simulink library "HIL_UDP_lib"  (Simulink 8.1)
settings: Solver=ode45  StartTime=0.0  StopTime=10.0  RelTol=1e-3
undefined symbols (not defined in the file): generic_ethernet_cb
libraries: HIL_UDP_lib x9, rtlab x2, simulink x2, opal_lib x1
settings Model: Creator=ch24070  LastModifiedBy=re25624

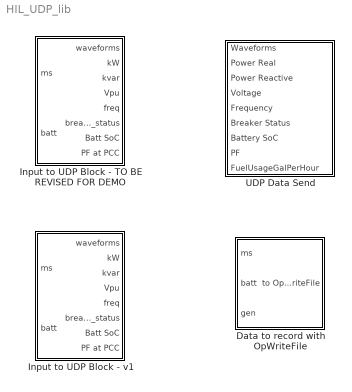
== system HIL_UDP_lib ==
  Data to record with OpWriteFile : Subsystem
  Input to UDP Block - TO BE REVISED FOR DEMO : Subsystem
  Input to UDP Block - v1 : Subsystem
  UDP Data Send : Subsystem

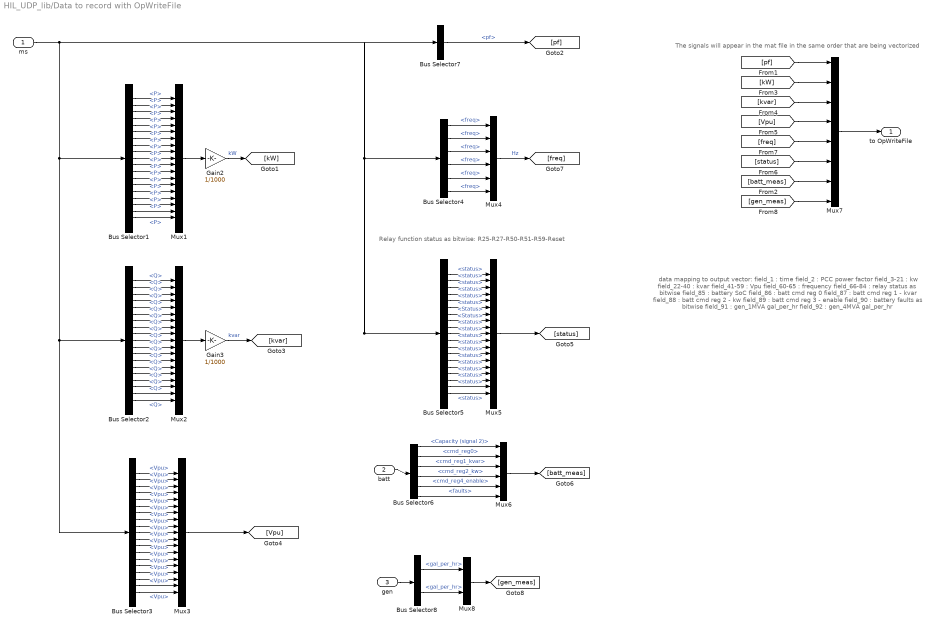
== system HIL_UDP_lib/Data to record with OpWriteFile ==
  note: The signals will appear in the mat file in the same order that are being vectorized
  note: Relay function status as bitwise:
      | R25-R27-R50-R51-R59-Reset
  note: data mapping to output vector:
      | field_1 : time
      | field_2 : PCC power factor
      | field_3-21 : kw
      | field_22-40 : kvar
      | field_41-59 : Vpu
      | field_60-65 : frequency
      | field_66-84 : relay status as bitwise
      | field_85 : battery SoC
      | field_86 : batt cmd reg 0
      | field_87 : batt cmd reg 1 - kvar
      | field_88 : batt cmd reg 2 - kw
      | field_89 : batt cmd reg 3 - enable
      | field_90 : battery faults as bitwise
      | field_91 : gen_1MVA gal_per_hr
      | field_92 : gen_4MVA gal_per_hr
  ms : Inport
  batt : Inport  Port=2
  gen : Inport  Port=3
  Bus Selector1 : BusSelector  OutputSignals=SEL_787_Relay1.m.P,SEL_787_Relay2.m.P,SEL_787_Relay3.m.P,SEL_787_Relay4.m.P,SEL_787_Relay5.m.P,SEL_787_Relay6.m.P,SEL_787_Relay7.P,SEL_787_Relay8.P,SEL_787_Relay9.m.P,SEL_787_Relay10.m.P,SEL_787_Relay11.m.P,SEL_787_Relay12.m.P,SEL_787_Relay13.m.P,SEL_787_Relay14.m.P,SEL_787_Relay15.m.P,SEL_787_Relay16.m.P,SEL_787_Relay17.m.P,SEL_787_Relay18.m.P,SEL_787_Relay19.m.P
  Bus Selector2 : BusSelector  OutputSignals=SEL_787_Relay1.m.Q,SEL_787_Relay2.m.Q,SEL_787_Relay3.m.Q,SEL_787_Relay4.m.Q,SEL_787_Relay5.m.Q,SEL_787_Relay6.m.Q,SEL_787_Relay7.Q,SEL_787_Relay8.Q,SEL_787_Relay9.m.Q,SEL_787_Relay10.m.Q,SEL_787_Relay11.m.Q,SEL_787_Relay12.m.Q,SEL_787_Relay13.m.Q,SEL_787_Relay14.m.Q,SEL_787_Relay15.m.Q,SEL_787_Relay16.m.Q,SEL_787_Relay17.m.Q,SEL_787_Relay18.m.Q,SEL_787_Relay19.m.Q
  Bus Selector3 : BusSelector  OutputSignals=SEL_787_Relay1.m.Vpu,SEL_787_Relay2.m.Vpu,SEL_787_Relay3.m.Vpu,SEL_787_Relay4.m.Vpu,SEL_787_Relay5.m.Vpu,SEL_787_Relay6.m.Vpu,SEL_787_Relay7.Vpu,SEL_787_Relay8.Vpu,SEL_787_Relay9.m.Vpu,SEL_787_Relay10.m.Vpu,SEL_787_Relay11.m.Vpu,SEL_787_Relay12.m.Vpu,SEL_787_Relay13.m.Vpu,SEL_787_Relay14.m.Vpu,SEL_787_Relay15.m.Vpu,SEL_787_Relay16.m.Vpu,SEL_787_Relay17.m.Vpu,SEL_787_Relay18.m.Vpu,SEL_787_Relay19.m.Vpu
  Bus Selector4 : BusSelector  OutputSignals=SEL_787_Relay1.m.freq,SEL_787_Relay3.m.freq,SEL_787_Relay7.freq,SEL_787_Relay8.freq,SEL_787_Relay13.m.freq,SEL_787_Relay17.m.freq
  Bus Selector5 : BusSelector  OutputSignals=SEL_787_Relay1.m.status,SEL_787_Relay2.m.status,SEL_787_Relay3.m.status,SEL_787_Relay4.m.status,SEL_787_Relay5.m.status,SEL_787_Relay6.m.status,SEL_787_Relay7.Status,SEL_787_Relay8.Status,SEL_787_Relay9.m.status,SEL_787_Relay10.m.status,SEL_787_Relay11.m.status,SEL_787_Relay12.m.status,SEL_787_Relay13.m.status,SEL_787_Relay14.m.status,SEL_787_Relay15.m.status,SEL_787_Relay16.m.status,SEL_787_Relay17.m.status,SEL_787_Relay18.m.status,SEL_787_Relay19.m.status
  Bus Selector6 : BusSelector  OutputSignals=Capacity.Capacity (signal 2),controller_cmds.cmd_reg0,controller_cmds.cmd_reg1_kvar,controller_cmds.cmd_reg2_kw,controller_cmds.cmd_reg4_enable,faults
  Bus Selector7 : BusSelector  OutputSignals=SEL_787_Relay1.m.pf
  Bus Selector8 : BusSelector  OutputSignals=gen_1MVA.gal_per_hr,gen_4MVA.gal_per_hr
  Gain2 : Gain  Gain=1/1000
  Gain3 : Gain  Gain=1/1000
  Mux{1..3,5} (4 alike) : Mux  Inputs=19
  Mux4 : Mux  Inputs=6
  Mux6 : Mux  Inputs=6
  Mux7 : Mux  Inputs=8
  Mux8 : Mux  Inputs=2
  to OpWriteFile : Outport
  wires:
  [gen_meas] -> Mux7/8
  Mux8/1 -> [gen_meas]
  Bus Selector8/2 -> Mux8/2  "<gal_per_hr>"
  Bus Selector8/1 -> Mux8/1  "<gal_per_hr>"
  gen/1 -> Bus Selector8/1
  Bus Selector4/6 -> Mux4/6  "<freq>"
  Bus Selector4/5 -> Mux4/5  "<freq>"
  Bus Selector4/4 -> Mux4/4  "<freq>"
  Bus Selector4/3 -> Mux4/3  "<freq>"
  Bus Selector4/2 -> Mux4/2  "<freq>"
  Bus Selector4/1 -> Mux4/1  "<freq>"
  Mux7/1 -> to OpWriteFile/1
  [batt_meas] -> Mux7/7
  [status] -> Mux7/6
  [freq] -> Mux7/5
  [Vpu] -> Mux7/4
  [kvar] -> Mux7/3
  [kW] -> Mux7/2
  [pf] -> Mux7/1
  Mux6/1 -> [batt_meas]
  Bus Selector6/6 -> Mux6/6  "<faults>"
  Bus Selector6/5 -> Mux6/5  "<cmd_reg4_enable>"
  Bus Selector6/4 -> Mux6/4  "<cmd_reg2_kw>"
  Bus Selector6/3 -> Mux6/3  "<cmd_reg1_kvar>"
  Bus Selector6/2 -> Mux6/2  "<cmd_reg0>"
  Bus Selector6/1 -> Mux6/1  "<Capacity (signal 2)>"
  Bus Selector7/1 -> [pf]  "<pf>"
  batt/1 -> Bus Selector6/1
  Bus Selector5/19 -> Mux5/19  "<status>"
  Bus Selector5/18 -> Mux5/18  "<status>"
  Bus Selector5/17 -> Mux5/17  "<status>"
  Bus Selector5/16 -> Mux5/16  "<status>"
  Bus Selector5/15 -> Mux5/15  "<status>"
  Bus Selector5/14 -> Mux5/14  "<status>"
  Bus Selector5/13 -> Mux5/13  "<status>"
  Bus Selector5/12 -> Mux5/12  "<status>"
  Bus Selector5/11 -> Mux5/11  "<status>"
  Bus Selector5/10 -> Mux5/10  "<status>"
  Bus Selector5/9 -> Mux5/9  "<status>"
  Bus Selector5/8 -> Mux5/8  "<Status>"
  Bus Selector5/7 -> Mux5/7  "<Status>"
  Bus Selector5/6 -> Mux5/6  "<status>"
  Bus Selector5/5 -> Mux5/5  "<status>"
  Bus Selector5/4 -> Mux5/4  "<status>"
  Bus Selector5/3 -> Mux5/3  "<status>"
  Bus Selector5/2 -> Mux5/2  "<status>"
  Bus Selector5/1 -> Mux5/1  "<status>"
  Mux5/1 -> [status]
  Mux4/1 -> [freq]  "Hz"
  Mux3/1 -> [Vpu]
  Bus Selector3/19 -> Mux3/19  "<Vpu>"
  Bus Selector3/18 -> Mux3/18  "<Vpu>"
  Bus Selector3/17 -> Mux3/17  "<Vpu>"
  Bus Selector3/16 -> Mux3/16  "<Vpu>"
  Bus Selector3/15 -> Mux3/15  "<Vpu>"
  Bus Selector3/14 -> Mux3/14  "<Vpu>"
  Bus Selector3/13 -> Mux3/13  "<Vpu>"
  Bus Selector3/12 -> Mux3/12  "<Vpu>"
  Bus Selector3/11 -> Mux3/11  "<Vpu>"
  Bus Selector3/10 -> Mux3/10  "<Vpu>"
  Bus Selector3/9 -> Mux3/9  "<Vpu>"
  Bus Selector3/8 -> Mux3/8  "<Vpu>"
  Bus Selector3/7 -> Mux3/7  "<Vpu>"
  Bus Selector3/6 -> Mux3/6  "<Vpu>"
  Bus Selector3/5 -> Mux3/5  "<Vpu>"
  Bus Selector3/4 -> Mux3/4  "<Vpu>"
  Bus Selector3/3 -> Mux3/3  "<Vpu>"
  Bus Selector3/2 -> Mux3/2  "<Vpu>"
  Bus Selector3/1 -> Mux3/1  "<Vpu>"
  Gain3/1 -> [kvar]  "kvar"
  Mux2/1 -> Gain3/1
  Bus Selector2/19 -> Mux2/19  "<Q>"
  Bus Selector2/18 -> Mux2/18  "<Q>"
  Bus Selector2/17 -> Mux2/17  "<Q>"
  Bus Selector2/16 -> Mux2/16  "<Q>"
  Bus Selector2/15 -> Mux2/15  "<Q>"
  Bus Selector2/14 -> Mux2/14  "<Q>"
  Bus Selector2/13 -> Mux2/13  "<Q>"
  Bus Selector2/12 -> Mux2/12  "<Q>"
  Bus Selector2/11 -> Mux2/11  "<Q>"
  Bus Selector2/10 -> Mux2/10  "<Q>"
  Bus Selector2/9 -> Mux2/9  "<Q>"
  Bus Selector2/8 -> Mux2/8  "<Q>"
  Bus Selector2/7 -> Mux2/7  "<Q>"
  Bus Selector2/6 -> Mux2/6  "<Q>"
  Bus Selector2/5 -> Mux2/5  "<Q>"
  Bus Selector2/4 -> Mux2/4  "<Q>"
  Bus Selector2/3 -> Mux2/3  "<Q>"
  Bus Selector2/2 -> Mux2/2  "<Q>"
  Bus Selector2/1 -> Mux2/1  "<Q>"
  Gain2/1 -> [kW]  "kW"
  Mux1/1 -> Gain2/1
  Bus Selector1/19 -> Mux1/19  "<P>"
  Bus Selector1/18 -> Mux1/18  "<P>"
  Bus Selector1/17 -> Mux1/17  "<P>"
  Bus Selector1/16 -> Mux1/16  "<P>"
  Bus Selector1/15 -> Mux1/15  "<P>"
  Bus Selector1/14 -> Mux1/14  "<P>"
  Bus Selector1/13 -> Mux1/13  "<P>"
  Bus Selector1/12 -> Mux1/12  "<P>"
  Bus Selector1/11 -> Mux1/11  "<P>"
  Bus Selector1/10 -> Mux1/10  "<P>"
  Bus Selector1/9 -> Mux1/9  "<P>"
  Bus Selector1/8 -> Mux1/8  "<P>"
  Bus Selector1/7 -> Mux1/7  "<P>"
  Bus Selector1/6 -> Mux1/6  "<P>"
  Bus Selector1/5 -> Mux1/5  "<P>"
  Bus Selector1/4 -> Mux1/4  "<P>"
  Bus Selector1/3 -> Mux1/3  "<P>"
  Bus Selector1/2 -> Mux1/2  "<P>"
  Bus Selector1/1 -> Mux1/1  "<P>"
  ms/1 -> Bus Selector7/1, Bus Selector5/1, Bus Selector4/1, Bus Selector3/1, Bus Selector2/1, Bus Selector1/1

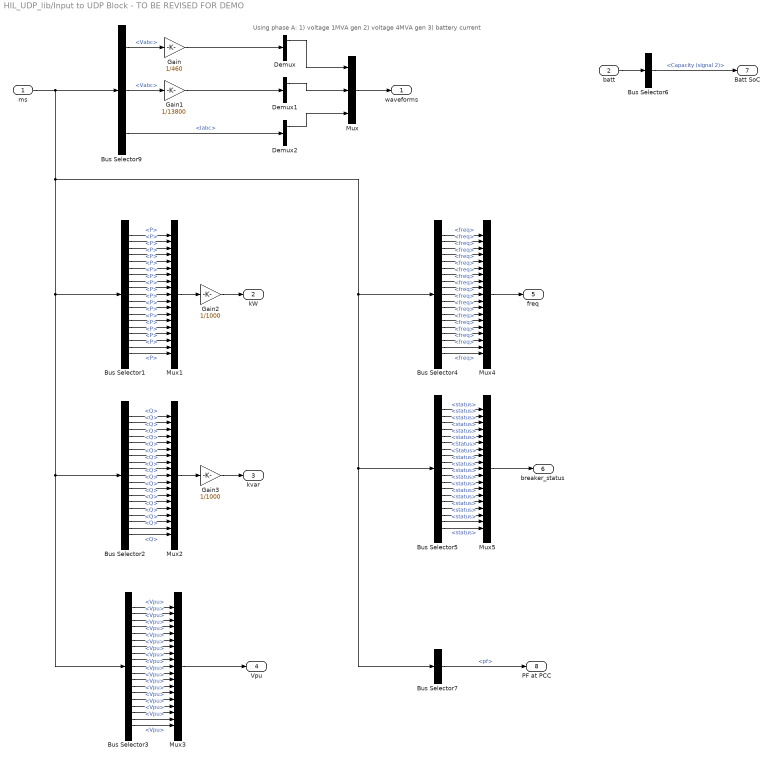
== system HIL_UDP_lib/Input to UDP Block - TO BE REVISED FOR DEMO ==
  note: Using phase A:
      | 1)  voltage 1MVA gen
      | 2) voltage 4MVA gen
      | 3) battery current
  ms : Inport
  batt : Inport  Port=2
  Bus Selector1 : BusSelector  OutputSignals=SEL_787_Relay1.m.P,SEL_787_Relay2.m.P,SEL_787_Relay3.m.P,SEL_787_Relay4.m.P,SEL_787_Relay5.m.P,SEL_787_Relay6.m.P,SEL_787_Relay7.P,SEL_787_Relay8.P,SEL_787_Relay9.m.P,SEL_787_Relay10.m.P,SEL_787_Relay11.m.P,SEL_787_Relay12.m.P,SEL_787_Relay13.m.P,SEL_787_Relay14.m.P,SEL_787_Relay15.m.P,SEL_787_Relay16.m.P,SEL_787_Relay17.m.P,SEL_787_Relay18.m.P,SEL_787_Relay19.m.P
  Bus Selector2 : BusSelector  OutputSignals=SEL_787_Relay1.m.Q,SEL_787_Relay2.m.Q,SEL_787_Relay3.m.Q,SEL_787_Relay4.m.Q,SEL_787_Relay5.m.Q,SEL_787_Relay6.m.Q,SEL_787_Relay7.Q,SEL_787_Relay8.Q,SEL_787_Relay9.m.Q,SEL_787_Relay10.m.Q,SEL_787_Relay11.m.Q,SEL_787_Relay12.m.Q,SEL_787_Relay13.m.Q,SEL_787_Relay14.m.Q,SEL_787_Relay15.m.Q,SEL_787_Relay16.m.Q,SEL_787_Relay17.m.Q,SEL_787_Relay18.m.Q,SEL_787_Relay19.m.Q
  Bus Selector3 : BusSelector  OutputSignals=SEL_787_Relay1.m.Vpu,SEL_787_Relay2.m.Vpu,SEL_787_Relay3.m.Vpu,SEL_787_Relay4.m.Vpu,SEL_787_Relay5.m.Vpu,SEL_787_Relay6.m.Vpu,SEL_787_Relay7.Vpu,SEL_787_Relay8.Vpu,SEL_787_Relay9.m.Vpu,SEL_787_Relay10.m.Vpu,SEL_787_Relay11.m.Vpu,SEL_787_Relay12.m.Vpu,SEL_787_Relay13.m.Vpu,SEL_787_Relay14.m.Vpu,SEL_787_Relay15.m.Vpu,SEL_787_Relay16.m.Vpu,SEL_787_Relay17.m.Vpu,SEL_787_Relay18.m.Vpu,SEL_787_Relay19.m.Vpu
  Bus Selector4 : BusSelector  OutputSignals=SEL_787_Relay1.m.freq,SEL_787_Relay2.m.freq,SEL_787_Relay3.m.freq,SEL_787_Relay4.m.freq,SEL_787_Relay5.m.freq,SEL_787_Relay6.m.freq,SEL_787_Relay7.freq,SEL_787_Relay8.freq,SEL_787_Relay9.m.freq,SEL_787_Relay10.m.freq,SEL_787_Relay11.m.freq,SEL_787_Relay12.m.freq,SEL_787_Relay13.m.freq,SEL_787_Relay14.m.freq,SEL_787_Relay15.m.freq,SEL_787_Relay16.m.freq,SEL_787_Relay17.m.freq,SEL_787_Relay18.m.freq,SEL_787_Relay19.m.freq
  Bus Selector5 : BusSelector  OutputSignals=SEL_787_Relay1.m.status,SEL_787_Relay2.m.status,SEL_787_Relay3.m.status,SEL_787_Relay4.m.status,SEL_787_Relay5.m.status,SEL_787_Relay6.m.status,SEL_787_Relay7.Status,SEL_787_Relay8.Status,SEL_787_Relay9.m.status,SEL_787_Relay10.m.status,SEL_787_Relay11.m.status,SEL_787_Relay12.m.status,SEL_787_Relay13.m.status,SEL_787_Relay14.m.status,SEL_787_Relay15.m.status,SEL_787_Relay16.m.status,SEL_787_Relay17.m.status,SEL_787_Relay18.m.status,SEL_787_Relay19.m.status
  Bus Selector6 : BusSelector  OutputSignals=Capacity.Capacity (signal 2)
  Bus Selector7 : BusSelector  OutputSignals=SEL_787_Relay1.m.pf
  Bus Selector9 : BusSelector  OutputSignals=SEL_787_Relay7.Vabc,SEL_787_Relay8.Vabc,SEL_787_Relay13.m.Iabc
  Demux : Demux  Outputs=3
  Demux1 : Demux  Outputs=3
  Demux2 : Demux  Outputs=3
  Gain : Gain  Gain=1/460
  Gain1 : Gain  Gain=1/13800
  Gain2 : Gain  Gain=1/1000
  Gain3 : Gain  Gain=1/1000
  Mux : Mux  Inputs=3
  Mux{1..5} (5 alike) : Mux  Inputs=19
  waveforms : Outport
  kW : Outport  Port=2
  kvar : Outport  Port=3
  Vpu : Outport  Port=4
  freq : Outport  Port=5
  breaker_status : Outport  Port=6
  Batt SoC : Outport  Port=7
  PF at PCC : Outport  Port=8
  wires:
  Bus Selector7/1 -> PF at PCC/1  "<pf>"
  Bus Selector6/1 -> Batt SoC/1  "<Capacity (signal 2)>"
  batt/1 -> Bus Selector6/1
  Bus Selector5/19 -> Mux5/19  "<status>"
  Bus Selector5/18 -> Mux5/18  "<status>"
  Bus Selector5/17 -> Mux5/17  "<status>"
  Bus Selector5/16 -> Mux5/16  "<status>"
  Bus Selector5/15 -> Mux5/15  "<status>"
  Bus Selector5/14 -> Mux5/14  "<status>"
  Bus Selector5/13 -> Mux5/13  "<status>"
  Bus Selector5/12 -> Mux5/12  "<status>"
  Bus Selector5/11 -> Mux5/11  "<status>"
  Bus Selector5/10 -> Mux5/10  "<status>"
  Bus Selector5/9 -> Mux5/9  "<status>"
  Bus Selector5/8 -> Mux5/8  "<Status>"
  Bus Selector5/7 -> Mux5/7  "<Status>"
  Bus Selector5/6 -> Mux5/6  "<status>"
  Bus Selector5/5 -> Mux5/5  "<status>"
  Bus Selector5/4 -> Mux5/4  "<status>"
  Bus Selector5/3 -> Mux5/3  "<status>"
  Bus Selector5/2 -> Mux5/2  "<status>"
  Bus Selector5/1 -> Mux5/1  "<status>"
  Mux5/1 -> breaker_status/1
  Bus Selector4/5 -> Mux4/5  "<freq>"
  Bus Selector4/4 -> Mux4/4  "<freq>"
  Bus Selector4/3 -> Mux4/3  "<freq>"
  Bus Selector4/2 -> Mux4/2  "<freq>"
  Bus Selector4/1 -> Mux4/1  "<freq>"
  Mux4/1 -> freq/1
  Mux3/1 -> Vpu/1
  Bus Selector3/19 -> Mux3/19  "<Vpu>"
  Bus Selector3/18 -> Mux3/18  "<Vpu>"
  Bus Selector3/17 -> Mux3/17  "<Vpu>"
  Bus Selector3/16 -> Mux3/16  "<Vpu>"
  Bus Selector3/15 -> Mux3/15  "<Vpu>"
  Bus Selector3/14 -> Mux3/14  "<Vpu>"
  Bus Selector3/13 -> Mux3/13  "<Vpu>"
  Bus Selector3/12 -> Mux3/12  "<Vpu>"
  Bus Selector3/11 -> Mux3/11  "<Vpu>"
  Bus Selector3/10 -> Mux3/10  "<Vpu>"
  Bus Selector3/9 -> Mux3/9  "<Vpu>"
  Bus Selector3/8 -> Mux3/8  "<Vpu>"
  Bus Selector3/7 -> Mux3/7  "<Vpu>"
  Bus Selector3/6 -> Mux3/6  "<Vpu>"
  Bus Selector3/5 -> Mux3/5  "<Vpu>"
  Bus Selector3/4 -> Mux3/4  "<Vpu>"
  Bus Selector3/3 -> Mux3/3  "<Vpu>"
  Bus Selector3/2 -> Mux3/2  "<Vpu>"
  Bus Selector3/1 -> Mux3/1  "<Vpu>"
  Gain3/1 -> kvar/1
  Mux2/1 -> Gain3/1
  Bus Selector2/19 -> Mux2/19  "<Q>"
  Bus Selector2/18 -> Mux2/18  "<Q>"
  Bus Selector2/17 -> Mux2/17  "<Q>"
  Bus Selector2/16 -> Mux2/16  "<Q>"
  Bus Selector2/15 -> Mux2/15  "<Q>"
  Bus Selector2/14 -> Mux2/14  "<Q>"
  Bus Selector2/13 -> Mux2/13  "<Q>"
  Bus Selector2/12 -> Mux2/12  "<Q>"
  Bus Selector2/11 -> Mux2/11  "<Q>"
  Bus Selector2/10 -> Mux2/10  "<Q>"
  Bus Selector2/9 -> Mux2/9  "<Q>"
  Bus Selector2/8 -> Mux2/8  "<Q>"
  Bus Selector2/7 -> Mux2/7  "<Q>"
  Bus Selector2/6 -> Mux2/6  "<Q>"
  Bus Selector2/5 -> Mux2/5  "<Q>"
  Bus Selector2/4 -> Mux2/4  "<Q>"
  Bus Selector2/3 -> Mux2/3  "<Q>"
  Bus Selector2/2 -> Mux2/2  "<Q>"
  Bus Selector2/1 -> Mux2/1  "<Q>"
  Gain2/1 -> kW/1
  Mux1/1 -> Gain2/1
  Bus Selector1/19 -> Mux1/19  "<P>"
  Bus Selector1/18 -> Mux1/18  "<P>"
  Bus Selector1/17 -> Mux1/17  "<P>"
  Bus Selector1/16 -> Mux1/16  "<P>"
  Bus Selector1/15 -> Mux1/15  "<P>"
  Bus Selector1/14 -> Mux1/14  "<P>"
  Bus Selector1/13 -> Mux1/13  "<P>"
  Bus Selector1/12 -> Mux1/12  "<P>"
  Bus Selector1/11 -> Mux1/11  "<P>"
  Bus Selector1/10 -> Mux1/10  "<P>"
  Bus Selector1/9 -> Mux1/9  "<P>"
  Bus Selector1/8 -> Mux1/8  "<P>"
  Bus Selector1/7 -> Mux1/7  "<P>"
  Bus Selector1/6 -> Mux1/6  "<P>"
  Bus Selector1/5 -> Mux1/5  "<P>"
  Bus Selector1/4 -> Mux1/4  "<P>"
  Bus Selector1/3 -> Mux1/3  "<P>"
  Bus Selector1/2 -> Mux1/2  "<P>"
  Bus Selector1/1 -> Mux1/1  "<P>"
  Mux/1 -> waveforms/1
  ms/1 -> Bus Selector7/1, Bus Selector5/1, Bus Selector4/1, Bus Selector3/1, Bus Selector2/1, Bus Selector1/1, Bus Selector9/1
  Gain1/1 -> Demux1/1
  Gain/1 -> Demux/1
  Demux2/1 -> Mux/3
  Demux/1 -> Mux/1
  Demux1/1 -> Mux/2
  Bus Selector9/2 -> Gain1/1  "<Vabc>"
  Bus Selector9/3 -> Demux2/1  "<Iabc>"
  Bus Selector9/1 -> Gain/1  "<Vabc>"
  Bus Selector4/6 -> Mux4/6  "<freq>"
  Bus Selector4/7 -> Mux4/7  "<freq>"
  Bus Selector4/8 -> Mux4/8  "<freq>"
  Bus Selector4/9 -> Mux4/9  "<freq>"
  Bus Selector4/10 -> Mux4/10  "<freq>"
  Bus Selector4/11 -> Mux4/11  "<freq>"
  Bus Selector4/12 -> Mux4/12  "<freq>"
  Bus Selector4/13 -> Mux4/13  "<freq>"
  Bus Selector4/14 -> Mux4/14  "<freq>"
  Bus Selector4/15 -> Mux4/15  "<freq>"
  Bus Selector4/16 -> Mux4/16  "<freq>"
  Bus Selector4/17 -> Mux4/17  "<freq>"
  Bus Selector4/18 -> Mux4/18  "<freq>"
  Bus Selector4/19 -> Mux4/19  "<freq>"

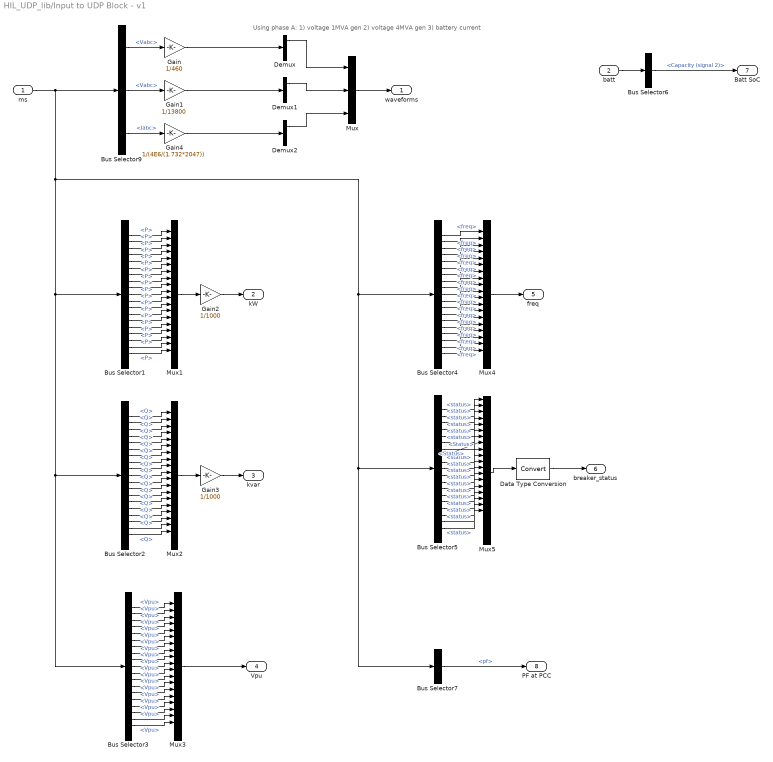
== system HIL_UDP_lib/Input to UDP Block - v1 ==
  note: Using phase A:
      | 1)  voltage 1MVA gen
      | 2) voltage 4MVA gen
      | 3) battery current
  ms : Inport
  batt : Inport  Port=2
  Bus Selector1 : BusSelector  OutputSignals=SEL_787_Relay1.m.P,SEL_787_Relay2.m.P,SEL_787_Relay3.m.P,SEL_787_Relay4.m.P,SEL_787_Relay5.m.P,SEL_787_Relay6.m.P,SEL_787_Relay7.P,SEL_787_Relay8.P,SEL_787_Relay9.m.P,SEL_787_Relay10.m.P,SEL_787_Relay11.m.P,SEL_787_Relay12.m.P,SEL_787_Relay13.m.P,SEL_787_Relay14.m.P,SEL_787_Relay15.m.P,SEL_787_Relay16.m.P,SEL_787_Relay17.m.P,SEL_787_Relay18.m.P,SEL_787_Relay19.m.P
  Bus Selector2 : BusSelector  OutputSignals=SEL_787_Relay1.m.Q,SEL_787_Relay2.m.Q,SEL_787_Relay3.m.Q,SEL_787_Relay4.m.Q,SEL_787_Relay5.m.Q,SEL_787_Relay6.m.Q,SEL_787_Relay7.Q,SEL_787_Relay8.Q,SEL_787_Relay9.m.Q,SEL_787_Relay10.m.Q,SEL_787_Relay11.m.Q,SEL_787_Relay12.m.Q,SEL_787_Relay13.m.Q,SEL_787_Relay14.m.Q,SEL_787_Relay15.m.Q,SEL_787_Relay16.m.Q,SEL_787_Relay17.m.Q,SEL_787_Relay18.m.Q,SEL_787_Relay19.m.Q
  Bus Selector3 : BusSelector  OutputSignals=SEL_787_Relay1.m.Vpu,SEL_787_Relay2.m.Vpu,SEL_787_Relay3.m.Vpu,SEL_787_Relay4.m.Vpu,SEL_787_Relay5.m.Vpu,SEL_787_Relay6.m.Vpu,SEL_787_Relay7.Vpu,SEL_787_Relay8.Vpu,SEL_787_Relay9.m.Vpu,SEL_787_Relay10.m.Vpu,SEL_787_Relay11.m.Vpu,SEL_787_Relay12.m.Vpu,SEL_787_Relay13.m.Vpu,SEL_787_Relay14.m.Vpu,SEL_787_Relay15.m.Vpu,SEL_787_Relay16.m.Vpu,SEL_787_Relay17.m.Vpu,SEL_787_Relay18.m.Vpu,SEL_787_Relay19.m.Vpu
  Bus Selector4 : BusSelector  OutputSignals=SEL_787_Relay1.m.freq,SEL_787_Relay2.m.freq,SEL_787_Relay3.m.freq,SEL_787_Relay4.m.freq,SEL_787_Relay5.m.freq,SEL_787_Relay6.m.freq,SEL_787_Relay7.freq,SEL_787_Relay8.freq,SEL_787_Relay9.m.freq,SEL_787_Relay10.m.freq,SEL_787_Relay11.m.freq,SEL_787_Relay12.m.freq,SEL_787_Relay13.m.freq,SEL_787_Relay14.m.freq,SEL_787_Relay15.m.freq,SEL_787_Relay16.m.freq,SEL_787_Relay17.m.freq,SEL_787_Relay18.m.freq,SEL_787_Relay19.m.freq
  Bus Selector5 : BusSelector  OutputSignals=SEL_787_Relay1.m.status,SEL_787_Relay2.m.status,SEL_787_Relay3.m.status,SEL_787_Relay4.m.status,SEL_787_Relay5.m.status,SEL_787_Relay6.m.status,SEL_787_Relay7.Status,SEL_787_Relay8.Status,SEL_787_Relay9.m.status,SEL_787_Relay10.m.status,SEL_787_Relay11.m.status,SEL_787_Relay12.m.status,SEL_787_Relay13.m.status,SEL_787_Relay14.m.status,SEL_787_Relay15.m.status,SEL_787_Relay16.m.status,SEL_787_Relay17.m.status,SEL_787_Relay18.m.status,SEL_787_Relay19.m.status
  Bus Selector6 : BusSelector  OutputSignals=Capacity.Capacity (signal 2)
  Bus Selector7 : BusSelector  OutputSignals=SEL_787_Relay1.m.pf
  Bus Selector9 : BusSelector  OutputSignals=SEL_787_Relay7.Vabc,SEL_787_Relay8.Vabc,SEL_787_Relay13.m.Iabc
  Data Type Conversion : DataTypeConversion
  Demux : Demux  Outputs=3
  Demux1 : Demux  Outputs=3
  Demux2 : Demux  Outputs=3
  Gain : Gain  Gain=1/460
  Gain1 : Gain  Gain=1/13800
  Gain2 : Gain  Gain=1/1000
  Gain3 : Gain  Gain=1/1000
  Gain4 : Gain  Gain=1/(4E6/(1.732*2047))
  Mux : Mux  Inputs=3
  Mux{1..4} (4 alike) : Mux  Inputs=20
  Mux5 : Mux  Inputs=24
  waveforms : Outport
  kW : Outport  Port=2
  kvar : Outport  Port=3
  Vpu : Outport  Port=4
  freq : Outport  Port=5
  breaker_status : Outport  Port=6
  Batt SoC : Outport  Port=7
  PF at PCC : Outport  Port=8
  wires:
  Bus Selector7/1 -> PF at PCC/1  "<pf>"
  Bus Selector6/1 -> Batt SoC/1  "<Capacity (signal 2)>"
  batt/1 -> Bus Selector6/1
  Bus Selector5/19 -> Mux5/19  "<status>"
  Bus Selector5/18 -> Mux5/18  "<status>"
  Bus Selector5/17 -> Mux5/17  "<status>"
  Bus Selector5/16 -> Mux5/16  "<status>"
  Bus Selector5/15 -> Mux5/15  "<status>"
  Bus Selector5/14 -> Mux5/14  "<status>"
  Bus Selector5/13 -> Mux5/13  "<status>"
  Bus Selector5/12 -> Mux5/12  "<status>"
  Bus Selector5/11 -> Mux5/11  "<status>"
  Bus Selector5/10 -> Mux5/10  "<status>"
  Bus Selector5/9 -> Mux5/9  "<status>"
  Bus Selector5/8 -> Mux5/8  "<Status>"
  Bus Selector5/7 -> Mux5/7  "<Status>"
  Bus Selector5/6 -> Mux5/6  "<status>"
  Bus Selector5/5 -> Mux5/5  "<status>"
  Bus Selector5/4 -> Mux5/4  "<status>"
  Bus Selector5/3 -> Mux5/3  "<status>"
  Bus Selector5/2 -> Mux5/2  "<status>"
  Bus Selector5/1 -> Mux5/1  "<status>"
  Mux5/1 -> Data Type Conversion/1
  Mux4/1 -> freq/1
  Mux3/1 -> Vpu/1
  Bus Selector3/19 -> Mux3/19  "<Vpu>"
  Bus Selector3/18 -> Mux3/18  "<Vpu>"
  Bus Selector3/17 -> Mux3/17  "<Vpu>"
  Bus Selector3/16 -> Mux3/16  "<Vpu>"
  Bus Selector3/15 -> Mux3/15  "<Vpu>"
  Bus Selector3/14 -> Mux3/14  "<Vpu>"
  Bus Selector3/13 -> Mux3/13  "<Vpu>"
  Bus Selector3/12 -> Mux3/12  "<Vpu>"
  Bus Selector3/11 -> Mux3/11  "<Vpu>"
  Bus Selector3/10 -> Mux3/10  "<Vpu>"
  Bus Selector3/9 -> Mux3/9  "<Vpu>"
  Bus Selector3/8 -> Mux3/8  "<Vpu>"
  Bus Selector3/7 -> Mux3/7  "<Vpu>"
  Bus Selector3/6 -> Mux3/6  "<Vpu>"
  Bus Selector3/5 -> Mux3/5  "<Vpu>"
  Bus Selector3/4 -> Mux3/4  "<Vpu>"
  Bus Selector3/3 -> Mux3/3  "<Vpu>"
  Bus Selector3/2 -> Mux3/2  "<Vpu>"
  Bus Selector3/1 -> Mux3/1  "<Vpu>"
  Gain3/1 -> kvar/1
  Mux2/1 -> Gain3/1
  Bus Selector2/19 -> Mux2/19  "<Q>"
  Bus Selector2/18 -> Mux2/18  "<Q>"
  Bus Selector2/17 -> Mux2/17  "<Q>"
  Bus Selector2/16 -> Mux2/16  "<Q>"
  Bus Selector2/15 -> Mux2/15  "<Q>"
  Bus Selector2/14 -> Mux2/14  "<Q>"
  Bus Selector2/13 -> Mux2/13  "<Q>"
  Bus Selector2/12 -> Mux2/12  "<Q>"
  Bus Selector2/11 -> Mux2/11  "<Q>"
  Bus Selector2/10 -> Mux2/10  "<Q>"
  Bus Selector2/9 -> Mux2/9  "<Q>"
  Bus Selector2/8 -> Mux2/8  "<Q>"
  Bus Selector2/7 -> Mux2/7  "<Q>"
  Bus Selector2/6 -> Mux2/6  "<Q>"
  Bus Selector2/5 -> Mux2/5  "<Q>"
  Bus Selector2/4 -> Mux2/4  "<Q>"
  Bus Selector2/3 -> Mux2/3  "<Q>"
  Bus Selector2/2 -> Mux2/2  "<Q>"
  Bus Selector2/1 -> Mux2/1  "<Q>"
  Gain2/1 -> kW/1
  Mux1/1 -> Gain2/1
  Bus Selector1/19 -> Mux1/19  "<P>"
  Bus Selector1/18 -> Mux1/18  "<P>"
  Bus Selector1/17 -> Mux1/17  "<P>"
  Bus Selector1/16 -> Mux1/16  "<P>"
  Bus Selector1/15 -> Mux1/15  "<P>"
  Bus Selector1/14 -> Mux1/14  "<P>"
  Bus Selector1/13 -> Mux1/13  "<P>"
  Bus Selector1/12 -> Mux1/12  "<P>"
  Bus Selector1/11 -> Mux1/11  "<P>"
  Bus Selector1/10 -> Mux1/10  "<P>"
  Bus Selector1/9 -> Mux1/9  "<P>"
  Bus Selector1/8 -> Mux1/8  "<P>"
  Bus Selector1/7 -> Mux1/7  "<P>"
  Bus Selector1/6 -> Mux1/6  "<P>"
  Bus Selector1/5 -> Mux1/5  "<P>"
  Bus Selector1/4 -> Mux1/4  "<P>"
  Bus Selector1/3 -> Mux1/3  "<P>"
  Bus Selector1/2 -> Mux1/2  "<P>"
  Bus Selector1/1 -> Mux1/1  "<P>"
  Mux/1 -> waveforms/1
  ms/1 -> Bus Selector7/1, Bus Selector5/1, Bus Selector4/1, Bus Selector3/1, Bus Selector2/1, Bus Selector1/1, Bus Selector9/1
  Gain1/1 -> Demux1/1
  Gain/1 -> Demux/1
  Demux2/1 -> Mux/3
  Demux/1 -> Mux/1
  Demux1/1 -> Mux/2
  Bus Selector9/2 -> Gain1/1  "<Vabc>"
  Bus Selector9/3 -> Gain4/1  "<Iabc>"
  Bus Selector9/1 -> Gain/1  "<Vabc>"
  Data Type Conversion/1 -> breaker_status/1
  Gain4/1 -> Demux2/1
  Bus Selector4/1 -> Mux4/1  "<freq>"
  Bus Selector4/2 -> Mux4/2  "<freq>"
  Bus Selector4/3 -> Mux4/3  "<freq>"
  Bus Selector4/4 -> Mux4/4  "<freq>"
  Bus Selector4/5 -> Mux4/5  "<freq>"
  Bus Selector4/6 -> Mux4/6  "<freq>"
  Bus Selector4/7 -> Mux4/7  "<freq>"
  Bus Selector4/8 -> Mux4/8  "<freq>"
  Bus Selector4/9 -> Mux4/9  "<freq>"
  Bus Selector4/10 -> Mux4/10  "<freq>"
  Bus Selector4/11 -> Mux4/11  "<freq>"
  Bus Selector4/12 -> Mux4/12  "<freq>"
  Bus Selector4/13 -> Mux4/13  "<freq>"
  Bus Selector4/14 -> Mux4/14  "<freq>"
  Bus Selector4/15 -> Mux4/15  "<freq>"
  Bus Selector4/16 -> Mux4/16  "<freq>"
  Bus Selector4/17 -> Mux4/17  "<freq>"
  Bus Selector4/18 -> Mux4/18  "<freq>"
  Bus Selector4/19 -> Mux4/19  "<freq>"

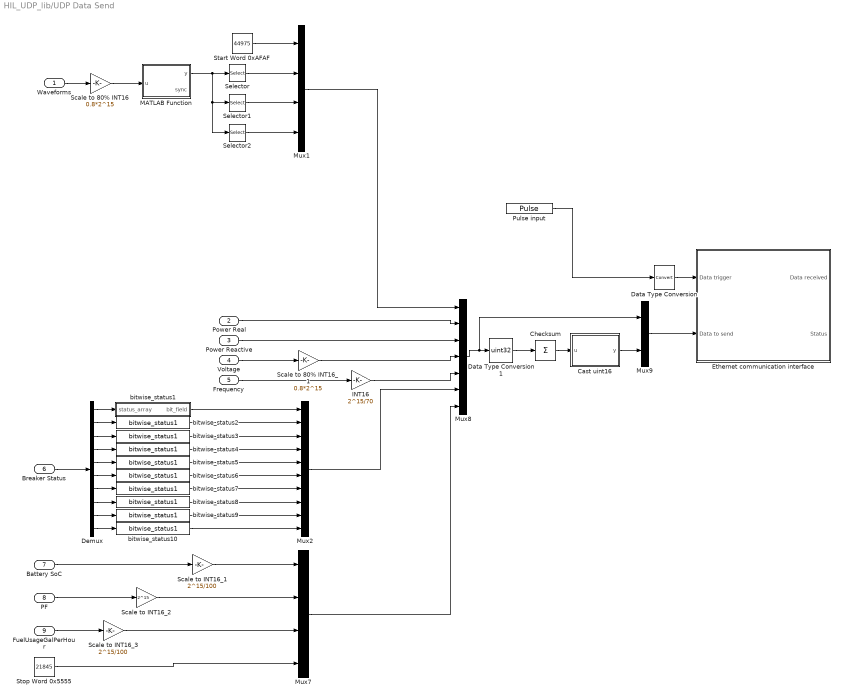
== system HIL_UDP_lib/UDP Data Send ==
  Waveforms : Inport  PortDimensions=3
  Power Real : Inport  Port=2  PortDimensions=20
  Power Reactive : Inport  Port=3  PortDimensions=20
  Voltage : Inport  Port=4  PortDimensions=20
  Frequency : Inport  Port=5  PortDimensions=20
  Breaker Status : Inport  Port=6  PortDimensions=20
  Battery SoC : Inport  Port=7  PortDimensions=1
  PF : Inport  Port=8  PortDimensions=1
  FuelUsageGalPerHour : Inport  Port=9  PortDimensions=2
  Cast uint16 : MATLAB Function  TreatAsAtomicUnit=on
  Checksum : Sum  Inputs=+
  Data Type Conversion : DataTypeConversion
  Data Type Conversion1 : DataTypeConversion  OutDataTypeStr=uint32  ConvertRealWorld=Stored Integer (SI)  RndMeth=Nearest
  Demux : Demux  Outputs=[2 2 2 2 2 2 2 2 2 2]
  Ethernet communication interface : Subsystem  mask(AsyncEthernet){ctrl_id=1, nbr_to_remote_endpoint=721, type_to_remote_endpoint=INT16, offset_to_remote_endpoint=0, swap_tx=off, nbr_from_remote_endpoint=4, type_from_remote_endpoint=UINT16, offset_from_remote_endpoint=0, swap_rx=off, exe_name='AsyncEthernet', nic_name='eth0', protocol=UDP, tcp_mode=Server, port=7200, remote_ip='255.255.255.255'}
      mask prompts: ctrl_id "Controller ID"; nbr_to_remote_endpoint "Number of data to send"; type_to_remote_endpoint "Type of data to send"; offset_to_remote_endpoint "Byte offset of transmission buffer"; swap_tx "Swap data endianness before transmission"; nbr_from_remote_endpoint "Number of data expected to be received"; type_from_remote_endpoint "Type of data expected to be received"; offset_from_remote_endpoint "Byte offset of reception buffer"; swap_rx "Swap data endianness after reception"; exe_name "Executable name"; nic_name "Network interface name"; tcp_mode "TCP mode"; port "Port number"; remote_ip "Remote IP address"
      mask help: This block is used as a communication interface to send data to a remote dedevice and receive data from it.
      mask Help: eval('rtlab_io_help(''Generic/Ethernet/Ethernet_interface.htm'');');
      mask Callback ctrl_id:
      | var = get_param(gcb,'ctrl_id');
      | set_param([gcb '/AsyncEthernetCtrl'],'ctrl_id',var)
      mask Callback nbr_to_remote_endpoint:
      | var = get_param(gcb,'nbr_to_remote_endpoint');
      | set_param([gcb '/AsyncEthernetCtrl'],'nbr_to_remote_endpoint',var)
      mask TypeOptions type_to_remote_endpoint: UINT8 | INT8 | UINT16 | INT16 | UINT32 | INT32 | FLOAT | DOUBLE
      mask Callback type_to_remote_endpoint:
      | var = get_param(gcb,'type_to_remote_endpoint');
      | set_param([gcb '/AsyncEthernetCtrl'],'type_to_remote_endpoint',var)
      mask Callback offset_to_remote_endpoint:
      | var = get_param(gcb,'offset_to_remote_endpoint');
      | set_param([gcb '/AsyncEthernetCtrl'],'offset_to_remote_endpoint',var)
      mask Callback swap_tx:
      | var = get_param(gcb,'swap_tx');
      | set_param([gcb '/AsyncEthernetCtrl'],'swap_tx',var)
      mask Callback nbr_from_remote_endpoint:
      | var = get_param(gcb,'nbr_from_remote_endpoint');
      | set_param([gcb '/AsyncEthernetCtrl'],'nbr_from_remote_endpoint',var)
      mask TypeOptions type_from_remote_endpoint: UINT8 | INT8 | UINT16 | INT16 | UINT32 | INT32 | FLOAT | DOUBLE
      mask Callback type_from_remote_endpoint:
      | var = get_param(gcb,'type_from_remote_endpoint');
      | set_param([gcb '/AsyncEthernetCtrl'],'type_from_remote_endpoint',var)
      mask Callback offset_from_remote_endpoint:
      | var = get_param(gcb,'offset_from_remote_endpoint');
      | set_param([gcb '/AsyncEthernetCtrl'],'offset_from_remote_endpoint',var)
      mask Callback swap_rx:
      | var = get_param(gcb,'swap_rx');
      | set_param([gcb '/AsyncEthernetCtrl'],'swap_rx',var)
      mask Callback exe_name:
      | str = get_param(gcb,'exe_name');
      | 
      | if exist('str','var')
      |     str = eval(str);
      | end
      | 
      | set_param([gcb '/AsyncEthernetCtrl'],'exe_name',str)
      mask Callback nic_name:
      | str = get_param(gcb,'nic_name');
      | 
      | if exist('str','var')
      |     str = eval(str);
      | end
      | 
      | set_param([gcb '/AsyncEthernetCtrl'],'nic_name',str)
      mask TypeOptions protocol: UDP | TCP
      mask Callback protocol: generic_ethernet_cb('protocol')
      mask TypeOptions tcp_mode: Client | Server
      mask Callback tcp_mode: generic_ethernet_cb('tcp_mode')
      mask Callback port:
      | var = get_param(gcb,'port');
      | set_param([gcb '/AsyncEthernetCtrl'],'port',var)
      mask Callback remote_ip:
      | str = get_param(gcb,'remote_ip');
      | 
      | if exist('str','var')
      |     str = eval(str);
      | end
      | 
      | set_param([gcb '/AsyncEthernetCtrl'],'remote_ip',str)
  INT16 : Gain  Gain=2^15/70
  MATLAB Function : MATLAB Function  TreatAsAtomicUnit=on
  Mux1 : Mux
  Mux2 : Mux  Inputs=10
  Mux7 : Mux
  Mux8 : Mux  Inputs=7
  Mux9 : Mux  Inputs=2
  Pulse input : DiscretePulseGenerator  PulseType=Time based  Period=1/5
  Scale to 80% INT16 : Gain  Gain=0.8*2^15
  Scale to 80% INT16_1 : Gain  Gain=0.8*2^15
  Scale to INT16_1 : Gain  Gain=2^15/100
  Scale to INT16_2 : Gain  Gain=2^15
  Scale to INT16_3 : Gain  Gain=2^15/100
  Selector : Selector  NumberOfDimensions=2  InputPortWidth=3  IndexOptions=Index vector (dialog),Select all  Indices=[1],1  OutputSizes=208,1
  Selector1 : Selector  NumberOfDimensions=2  InputPortWidth=3  IndexOptions=Index vector (dialog),Select all  Indices=[2],1  OutputSizes=208,1
  Selector2 : Selector  NumberOfDimensions=2  InputPortWidth=3  IndexOptions=Index vector (dialog),Select all  Indices=[3],1  OutputSizes=208,1
  Start Word 0xAFAF : Constant  Value=44975  OutDataTypeStr=double
  Stop Word 0x5555 : Constant  Value=21845  OutDataTypeStr=double
  bitwise_status1 : Subsystem
  bitwise_status{2..10} (9 alike) : HIL_UDP_lib/UDP Data Send/bitwise_status1
  wires:
  Start Word 0xAFAF/1 -> Mux1/1
  Pulse input/1 -> Data Type Conversion/1
  Data Type Conversion/1 -> Ethernet communication interface/1(Data trigger)
  Waveforms/1 -> Scale to 80% INT16/1
  MATLAB Function/1(y) -> Selector/1, Selector1/1, Selector2/1
  Selector/1 -> Mux1/2
  Selector1/1 -> Mux1/3
  Selector2/1 -> Mux1/4
  Mux1/1 -> Mux8/1
  Mux8/1 -> Mux9/1, Data Type Conversion1/1
  Checksum/1 -> Cast uint16/1(u)
  Cast uint16/1(y) -> Mux9/2
  Mux9/1 -> Ethernet communication interface/2(Data to send)
  Power Real/1 -> Mux8/2
  Power Reactive/1 -> Mux8/3
  Voltage/1 -> Scale to 80% INT16_1/1
  Frequency/1 -> INT16/1
  Demux/1 -> bitwise_status1/1(status_array)
  Breaker Status/1 -> Demux/1
  Data Type Conversion1/1 -> Checksum/1
  Battery SoC/1 -> Scale to INT16_1/1
  PF/1 -> Scale to INT16_2/1
  Scale to 80% INT16_1/1 -> Mux8/4
  INT16/1 -> Mux8/5
  FuelUsageGalPerHour/1 -> Scale to INT16_3/1
  Stop Word 0x5555/1 -> Mux7/4
  Scale to INT16_1/1 -> Mux7/1
  Scale to INT16_2/1 -> Mux7/2
  Scale to INT16_3/1 -> Mux7/3
  Mux2/1 -> Mux8/6
  Mux7/1 -> Mux8/7
  bitwise_status1/1(bit_field) -> Mux2/1
  Demux/2 -> bitwise_status2/1
  Demux/3 -> bitwise_status3/1
  Demux/4 -> bitwise_status4/1
  Demux/5 -> bitwise_status5/1
  Demux/6 -> bitwise_status6/1
  Demux/7 -> bitwise_status7/1
  Demux/8 -> bitwise_status8/1
  Demux/9 -> bitwise_status9/1
  Demux/10 -> bitwise_status10/1
  bitwise_status2/1 -> Mux2/2
  bitwise_status3/1 -> Mux2/3
  bitwise_status4/1 -> Mux2/4
  bitwise_status5/1 -> Mux2/5
  bitwise_status6/1 -> Mux2/6
  bitwise_status7/1 -> Mux2/7
  bitwise_status8/1 -> Mux2/8
  bitwise_status9/1 -> Mux2/9
  bitwise_status10/1 -> Mux2/10
  Scale to 80% INT16/1 -> MATLAB Function/1(u)

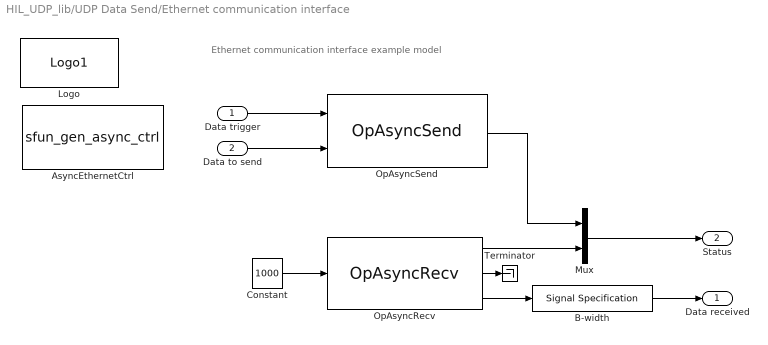
== system HIL_UDP_lib/UDP Data Send/Ethernet communication interface ==
  note: Ethernet communication interface example model
  Data trigger : Inport
  Data to send : Inport  Port=2
  AsyncEthernetCtrl : S-Function  InitFcn=generic_ethernet_cb('initfcn');  FunctionName=sfun_gen_async_ctrl  Parameters=ctrl_id, nbr_to_remote_endpoint, type_to_remote_endpoint,nbr_from_remote_endpoint,type_from_remote_endpoint,protocol,tcp_mode, port, offset_to_remote_endpoint,offset_from_remote_endpoint,swap_tx,swap_rx,0,nic_name,remote_ip,'','','','','','','','','','',exe_name,0  EnableBusSupport=off  mask(AsyncEthernetCtrl){ctrl_id=1, nbr_to_remote_endpoint=721, type_to_remote_endpoint=INT16, offset_to_remote_endpoint=0, nbr_from_remote_endpoint=4, type_from_remote_endpoint=UINT16, offset_from_remote_endpoint=0, nic_name=eth0, protocol=UDP, tcp_mode=Server, port=7200, remote_ip=255.255.255.255, exe_name=AsyncEthernet, swap_tx=off, swap_rx=off}
      mask prompts: ctrl_id "Controller ID"; nbr_to_remote_endpoint "Number of data to send"; type_to_remote_endpoint "Type of data to send"; offset_to_remote_endpoint "Byte offset of transmission buffer"; nbr_from_remote_endpoint "Number of data expected to be received"; type_from_remote_endpoint "Type of data expected to be received"; offset_from_remote_endpoint "Byte offset of reception buffer"; nic_name "Network interface name"; tcp_mode "TCP mode"; remote_ip "Remote IP address"; exe_name "Name of the executable"; swap_tx "Swap data endianness before transmission"; swap_rx "Swap data endianness after reception"
      mask help: Generic asynchronous process configuration block
      mask Help: eval('rtlab_help(''opasyncgenctrl'');');
      mask TypeOptions type_to_remote_endpoint: UINT8 | INT8 | UINT16 | INT16 | UINT32 | INT32 | FLOAT | DOUBLE
      mask TypeOptions type_from_remote_endpoint: UINT8 | INT8 | UINT16 | INT16 | UINT32 | INT32 | FLOAT | DOUBLE
      mask TypeOptions protocol: UDP | TCP
      mask TypeOptions tcp_mode: Client | Server
      mask Display: disp(sprintf('\nEthernet communication \ninterface controller\n'))
  B-width : SignalSpecification  Dimensions=nbr_from_remote_endpoint
  Constant : Constant  Value=1000
  Logo : opal_lib/Logo1  vide=[]
  Mux : Mux  Inputs=2
  OpAsyncRecv : rtlab/Communication/Asynchronous/OpAsyncRecv  ctl_id=ctrl_id  recv_id=ctrl_id  enable_param=off  fp1=1  fp2=2  fp3=3  fp4=4  fp5=5  sp1=string1  sp2=string2  sp3=string3  sp4=string4  sp5=string5
  OpAsyncSend : rtlab/Communication/Asynchronous/OpAsyncSend  ctl_id=ctrl_id  send_id=ctrl_id  mode=DONT_NEED_REPLY  enable_param=off  fp1=1  fp2=2  fp3=3  fp4=4  fp5=5  sp1=string1  sp2=string2  sp3=string3  sp4=string4  sp5=string5
  Terminator : Terminator
  Data received : Outport
  Status : Outport  Port=2
  wires:
  B-width/1 -> Data received/1
  OpAsyncRecv/3 -> B-width/1
  OpAsyncRecv/2 -> Terminator/1
  Constant/1 -> OpAsyncRecv/1
  Mux/1 -> Status/1
  OpAsyncRecv/1 -> Mux/2
  OpAsyncSend/1 -> Mux/1
  Data trigger/1 -> OpAsyncSend/1
  Data to send/1 -> OpAsyncSend/2

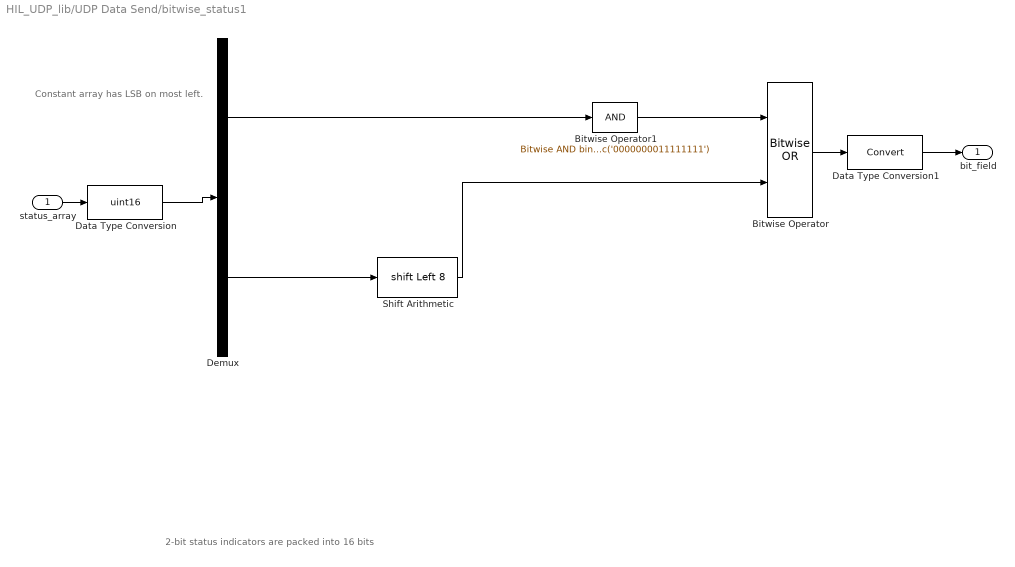
== system HIL_UDP_lib/UDP Data Send/bitwise_status1 ==
  note: Constant array has LSB on most left.
  note: 2-bit status indicators are packed into 16 bits
  status_array : Inport
  Bitwise Operator : simulink/Logic and Bit Operations/Bitwise Operator  logicop=OR  UseBitMask=off  NumInputPorts=2  BitMask=bin2dec('11011001')  BitMaskRealWorld=Stored Integer
  Bitwise Operator1 : simulink/Logic and Bit Operations/Bitwise Operator  logicop=AND  UseBitMask=on  BitMask=bin2dec('0000000011111111')  BitMaskRealWorld=Stored Integer
  Data Type Conversion : DataTypeConversion  OutDataTypeStr=uint16
  Data Type Conversion1 : DataTypeConversion
  Demux : Demux  Outputs=2
  Shift Arithmetic : ArithShift  BitShiftNumber=8  BitShiftDirection=Left
  bit_field : Outport
  wires:
  Data Type Conversion1/1 -> bit_field/1
  Bitwise Operator/1 -> Data Type Conversion1/1
  status_array/1 -> Data Type Conversion/1
  Demux/2 -> Shift Arithmetic/1
  Demux/1 -> Bitwise Operator1/1
  Data Type Conversion/1 -> Demux/1
  Shift Arithmetic/1 -> Bitwise Operator/2
  Bitwise Operator1/1 -> Bitwise Operator/1

== matlab function UDP Data Send/Cast uint16 ==
  data: u input double; y output double
function y = fcn(u)
%#codegen

x = double(typecast(uint32(u),'uint16'));
y = x(1); % low bits

== matlab function UDP Data Send/MATLAB Function ==
  data: u input double; y output double; sync output double
function [y, sync] = fcn(u)
%#codegen

[y, sync] = scopeBuffer(u);
